simulink model "prob_1"  (R2019b)
settings: Solver=VariableStepAuto  StartTime=0.0  StopTime=10.0  RelTol=1e-3
settings Model: Creator=kcalp  LastModifiedBy=kcalp

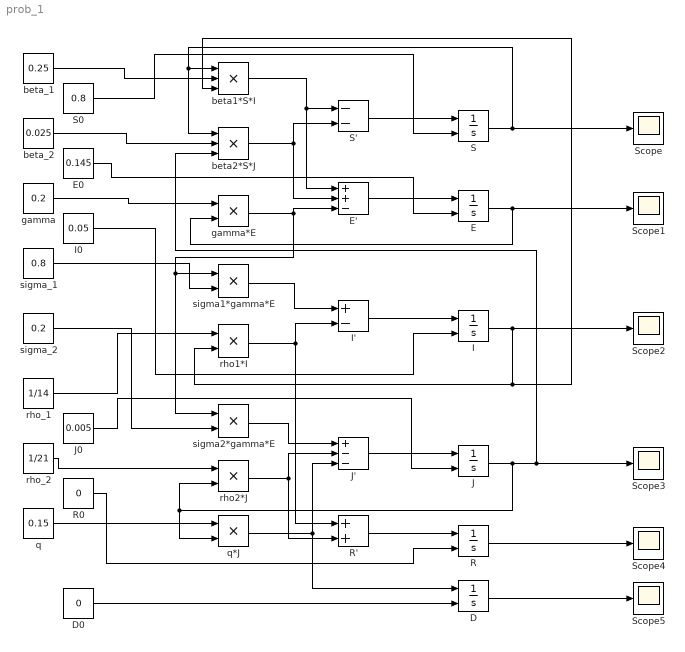
== system prob_1 ==
  D : Integrator  InitialConditionSource=external
  D0 : Constant  Value=0
  E : Integrator  InitialConditionSource=external
  "E' " : Sum  Inputs=++-
  "E0 " : Constant  Value=0.145
  "I " : Integrator  InitialConditionSource=external
  "I' " : Sum  Inputs=+-
  "I0 " : Constant  Value=0.05
  J : Integrator  InitialConditionSource=external
  "J' " : Sum  Inputs=+--
  "J0 " : Constant  Value=0.005
  R : Integrator  InitialConditionSource=external
  "R' " : Sum  Inputs=2
  R0 : Constant  Value=0
  S : Integrator  InitialConditionSource=external
  "S' " : Sum  Inputs=--
  "S0 " : Constant  Value=0.8
  Scope{,1..5} (6 alike) : Scope
  "beta1*S*I " : Product  Inputs=3
  beta2*S*J : Product  Inputs=3
  "beta_1 " : Constant  Value=0.25
  "beta_2 " : Constant  Value=0.025
  "gamma " : Constant  Value=0.2
  "gamma*E " : Product
  q : Constant  Value=0.15
  q*J : Product
  rho1*I : Product
  rho2*J : Product
  rho_1 : Constant  Value=1/14
  "rho_2 " : Constant  Value=1/21
  "sigma1*gamma*E " : Product
  "sigma2*gamma*E " : Product
  sigma_1 : Constant  Value=0.8
  sigma_2 : Constant  Value=0.2
  wires:
  "beta1*S*I "/1 -> "E' "/1, "S' "/1
  beta2*S*J/1 -> "S' "/2, "E' "/2
  "S0 "/1 -> S/2
  "S' "/1 -> S/1
  "beta_1 "/1 -> "beta1*S*I "/2
  "beta_2 "/1 -> beta2*S*J/2
  S/1 -> Scope/1, "beta1*S*I "/1, beta2*S*J/1
  "gamma "/1 -> "gamma*E "/1
  E/1 -> Scope1/1, "gamma*E "/2
  "gamma*E "/1 -> "sigma1*gamma*E "/1, "sigma2*gamma*E "/1, "E' "/3
  "E' "/1 -> E/1
  "E0 "/1 -> E/2
  sigma_1/1 -> "sigma1*gamma*E "/2
  "sigma1*gamma*E "/1 -> "I' "/1
  rho1*I/1 -> "R' "/1, "I' "/2
  "I' "/1 -> "I "/1
  "I0 "/1 -> "I "/2
  "I "/1 -> "beta1*S*I "/3, rho1*I/2, Scope2/1
  rho_1/1 -> rho1*I/1
  sigma_2/1 -> "sigma2*gamma*E "/2
  J/1 -> beta2*S*J/3, Scope3/1, rho2*J/2, q*J/2
  "sigma2*gamma*E "/1 -> "J' "/1
  "J' "/1 -> J/1
  "J0 "/1 -> J/2
  "R' "/1 -> R/1
  R0/1 -> R/2
  R/1 -> Scope4/1
  q/1 -> q*J/1
  "rho_2 "/1 -> rho2*J/1
  rho2*J/1 -> "J' "/2, "R' "/2
  q*J/1 -> "J' "/3, D/1
  D0/1 -> D/2
  D/1 -> Scope5/1
